simulink model "Assignment1"  (R2022a)
settings: Solver=VariableStepAuto  StartTime=0.0  StopTime=10.0  RelTol=1e-3
settings Model: Creator=keryn  LastModifiedBy=keryn

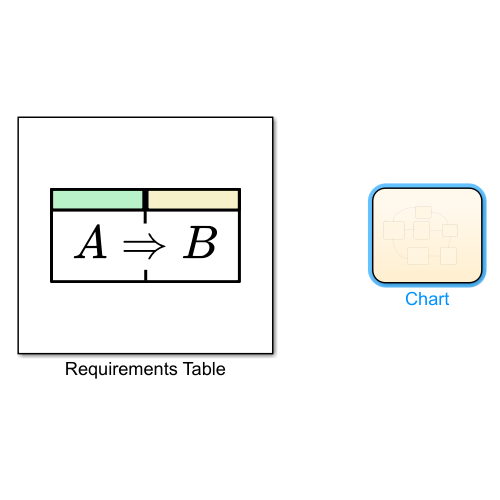
[thumbnail: Simulink's stored preview of the top-level diagram]
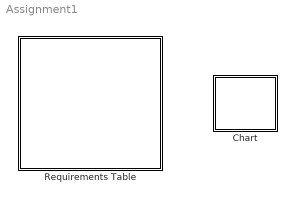
== system Assignment1 ==
  Chart : Stateflow chart  TreatAsAtomicUnit=on
  Requirements Table : Requirements Table  TreatAsAtomicUnit=on

== stateflow chart Assignment1/Requirements Table ==
  (default) -> (junction 1073741860)
  (junction 1073741860) -> (junction 1073741861) : {
      | % SF_REQ_REV_07
      | }
  (junction 1073741861) -> (junction 1073741863) : {
      | % HEADER_ASSIGNMENTS
      |
      | }
  (junction 1073741863) -> (junction 1073741865) : {
      | % START_A_4
      | }
  (junction 1073741865) -> (junction 1073741867) : {
      | }
  (junction 1073741867) -> (junction 1073741869)
  (junction 1073741869) -> (junction 1073741871) : {
      | }
  (junction 1073741871) -> (junction 1073741873) : {
      | % END_A_4
      | }
  (junction 1073741873) -> (junction 1073741898) : {
      | % START_R_1
      | }
  (junction 1073741898) -> (junction 1073741900) : {
      | }
  (junction 1073741900) -> (junction 1073741902) : {
      |
      |
      | }
  (junction 1073741902) -> (junction 1073741904) : {
      | }
  (junction 1073741904) -> (junction 1073741906) : {
      | % END_R_1
      | }

== stateflow chart Assignment1/Chart ==
  state Natural_Pulse
    entry:
    FRONTEND_CTRL = LOW;
    %turn off sensor
  state VVI_Initial_State
    entry:
    FRONTEND_CTRL= HIGH;
    %sensing open
    Z_ATR_CTRL = LOW;
    Z_VENT_CTRL = LOW;
    %defult setting
    PACE_GND_CTRL = HIGH;
    VENT_GND_CTRL = HIGH;
    %VENT_CMP_REF_PWM = 70;
    %discharging C21
    PACING_REF_PWM = ATR_AMP*20;
    %setting pacing amplitude
    NATURAL_PULSE = LOW;
    RED_LED = LOW;
    %assuming no natural pulse as defalt
  state VVI_Charging_State
    entry:
    ATR_PACE_CTRL = LOW;
    VENT_PACE_CTRL = LOW;
    PACE_CHARGE_CTRL = HIGH;
    PACING_REF_PWM = ATR_AMP*20;
    %setting pacing amplitude
    %charge C22
    RED_LED = HIGH;
    %show us it is charging
  state Checking_state
    entry:
    PACING_REF_PWM = ATR_AMP*20;
    %setting pacing amplitude
    %Is this state necessary?
  state Discharge_State
    entry:
    PACE_GND_CTRL = HIGH;
    VENT_PACE_CTRL = LOW;
    Z_ATR_CTRL = LOW;
    Z_VENT_ CTRL = LOW;
    ATR_PACE_CTRL = LOW;
    ATR_GND_CTRL = LOW;
    VENT_GND_CTRL = HIGH;
    %dischaging C21
    FRONTEND_CTRL = LOW;
  state Pacing_State
    entry:
    PACE_CHARGE_CTRL = LOW;
    PACE_GND_CTRL = HIGH;
    ATR_PACE_CTRL = LOW;
    ATR_GND_CTRL = LOW;
    Z_ATR_CTRL = LOW;
    Z_VENT_CTRL = LOW;
    VENT_GND_CTRL = LOW;
    VENT_PACE_CTRL = HIGH;
    %PACING_REF_PWM = ATR_AMP*20;
  Natural_Pulse -> VVI_Initial_State
  Checking_state -> Natural_Pulse [order 1] : [VENT_CMP_DETECT == HIGH]
  (default) -> VVI_Initial_State
  VVI_Initial_State -> VVI_Charging_State
  VVI_Charging_State -> Checking_state : [after(Vent_Refractory,msec)]
  Checking_state -> Pacing_State [order 2] : [after(60000/LRL - Vent_Refractory - Pulse_width, msec)]
  Discharge_State -> VVI_Initial_State
  Pacing_State -> Discharge_State : [after(Pulse_Width,msec)]
